simulink model "hexa_quaternion_FxTESO_ANSFT"  (R2023a)
settings: Solver=ode4  StartTime=0.0  StopTime=60  FixedStep=0.01  RelTol=1e-3
undefined symbols (not defined in the file or in its folder): F, Light, MIL
libraries: sharedtransform x9, dspsrcs4 x9, aerolibutil x8, simulink x5, sharedutil x3, simulink_extras x3, matrix_library x2, robotcorelib x1, aerolibwind2 x1, uavutilslib x1
(part 2 of 2)

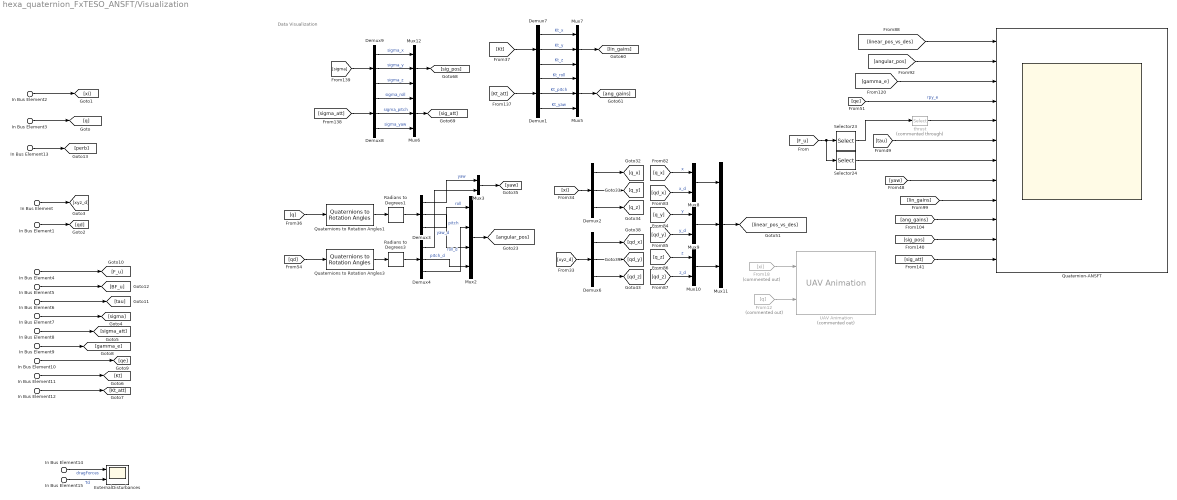
== system hexa_quaternion_FxTESO_ANSFT/Visualization ==
  note: Data Visualization
  In Bus Element2 : Inport  PortName=gamma_eta  Element=x
  In Bus Element3 : Inport  PortName=gamma_eta  Element=q
  In Bus Element13 : Inport  PortName=gamma_eta  Element=perb
  In Bus Element : Inport  Port=2  PortName=gamma_eta_d  Element=xyz_d
  In Bus Element1 : Inport  Port=2  PortName=gamma_eta_d  Element=qd
  In Bus Element4 : Inport  Port=3  PortName=u  Element=F_u
  In Bus Element5 : Inport  Port=3  PortName=u  Element=B-F_u
  In Bus Element6 : Inport  Port=3  PortName=u  Element=tau
  In Bus Element7 : Inport  Port=3  PortName=u  Element=sigma
  In Bus Element8 : Inport  Port=3  PortName=u  Element=sigma_att
  In Bus Element9 : Inport  Port=3  PortName=u  Element=gamma_e
  In Bus Element10 : Inport  Port=3  PortName=u  Element=eta_e
  In Bus Element11 : Inport  Port=3  PortName=u  Element=Kt
  In Bus Element12 : Inport  Port=3  PortName=u  Element=Kt_att
  In Bus Element14 : Inport  Port=4  PortName=perb  Element=perb
  In Bus Element15 : Inport  Port=4  PortName=perb  Element=Td
  Demux{1..4,6..9} (8 alike) : Demux  Outputs=3
  ExternalDisturbances : Scope  NumInputPorts=2
  From12 : From  Commented=on  GotoTag=q
  From18 : From  Commented=on  GotoTag=xi
  Mux{3,8..10} (4 alike) : Mux  Inputs=2
  Mux{5..7,11..12} (5 alike) : Mux  Inputs=3
  Mux2 : Mux
  Quaternion-ANSFT : Scope  NumInputPorts=12
  Quaternions to Rotation Angles1 : sharedtransform/Quaternions to Rotation Angles  rotationOrder=ZYX  aMode=aMode
  Quaternions to Rotation Angles3 : sharedtransform/Quaternions to Rotation Angles  rotationOrder=ZYX  aMode=aMode
  Radians to Degrees1 : simulink_extras/Transformations/Radians to Degrees
  Radians to Degrees3 : simulink_extras/Transformations/Radians to Degrees
  Selector23 : Selector  InputPortWidth=3  IndexOptions=Index vector (dialog)  Indices=[3]  OutputSizes=1
  Selector24 : Selector  InputPortWidth=3  IndexOptions=Index vector (dialog)  Indices=[1:2]  OutputSizes=1
  UAV Animation : uavutilslib/UAV Animation  Commented=on  UAVType=Multirotor  UAVSize=1  InertialZDirection=Down  SampleTime=-1
  thrust : Selector  Commented=through  InputPortWidth=3  IndexOptions=Index vector (dialog)  Indices=[3]  OutputSizes=1
  wires:
  [sigma_att] -> Demux8/1
  Radians to Degrees1/1 -> Demux3/1
  Demux3/3 -> Mux2/1  "roll"
  [lin_gains] -> Quaternion-ANSFT/9
  Mux11/1 -> [linear_pos_vs_des]
  [qe] -> Quaternion-ANSFT/4  "rpy_e"
  Mux3/1 -> [yaw]
  Demux6/1 -> [qd_x]
  Demux9/2 -> Mux12/2  "sigma_y"
  [yaw] -> Quaternion-ANSFT/8
  Mux5/1 -> [ang_gains]
  Mux10/1 -> Mux11/3
  Demux1/1 -> Mux5/1  "Kt_roll"
  Demux7/3 -> Mux7/3  "Kt_z"
  From12/1 -> UAV Animation/2
  [q_z] -> Mux10/1  "z"
  [linear_pos_vs_des] -> Quaternion-ANSFT/1
  Quaternions to Rotation Angles1/1 -> Radians to Degrees1/1
  [Kt] -> Demux7/1
  Demux4/2 -> Mux2/4  "pitch_d"
  Demux7/1 -> Mux7/1  "Kt_x"
  [qd] -> Quaternions to Rotation Angles3/1
  [qd_x] -> Mux8/2  "x_d"
  Demux7/2 -> Mux7/2  "Kt_y"
  Mux7/1 -> [lin_gains]
  Demux8/3 -> Mux6/3  "sigma_yaw"
  Demux6/2 -> [qd_y]
  [xyz_d] -> Demux6/1
  [gamma_e] -> Quaternion-ANSFT/3
  [sig_att] -> Quaternion-ANSFT/12
  [F_u] -> Selector24/1, Selector23/1
  Demux4/1 -> Mux3/2  "yaw_d"
  Selector24/1 -> Quaternion-ANSFT/7
  [q_x] -> Mux8/1  "x"
  [ang_gains] -> Quaternion-ANSFT/10
  Demux1/3 -> Mux5/3  "Kt_yaw"
  Mux9/1 -> Mux11/2
  Selector23/1 -> thrust/1
  Demux2/3 -> [q_z]
  Mux8/1 -> Mux11/1
  Demux3/1 -> Mux3/1  "yaw"
  [sig_pos] -> Quaternion-ANSFT/11
  [tau] -> Quaternion-ANSFT/6
  From18/1 -> UAV Animation/1
  Quaternions to Rotation Angles3/1 -> Radians to Degrees3/1
  Demux6/3 -> [qd_z]
  [q] -> Quaternions to Rotation Angles1/1
  Radians to Degrees3/1 -> Demux4/1
  [qd_z] -> Mux10/2  "z_d"
  Demux1/2 -> Mux5/2  "Kt_pitch"
  [qd_y] -> Mux9/2  "y_d"
  thrust/1 -> Quaternion-ANSFT/5
  Mux12/1 -> [sig_pos]
  Mux6/1 -> [sig_att]
  Demux2/2 -> [q_y]
  [sigma] -> Demux9/1
  Demux9/3 -> Mux12/3  "sigma_z"
  [q_y] -> Mux9/1  "y"
  Demux8/2 -> Mux6/2  "sigma_pitch"
  Demux2/1 -> [q_x]
  [Kt_att] -> Demux1/1
  Demux3/2 -> Mux2/3  "pitch"
  Mux2/1 -> [angular_pos]
  Demux9/1 -> Mux12/1  "sigma_x"
  Demux8/1 -> Mux6/1  "sigma_roll"
  [xi] -> Demux2/1
  [angular_pos] -> Quaternion-ANSFT/2
  Demux4/3 -> Mux2/2  "roll_d"
  In Bus Element3/1 -> [q]
  In Bus Element2/1 -> [xi]
  In Bus Element1/1 -> [qd]
  In Bus Element/1 -> [xyz_d]
  In Bus Element6/1 -> [tau]
  In Bus Element7/1 -> [sigma]
  In Bus Element8/1 -> [sigma_att]
  In Bus Element9/1 -> [gamma_e]
  In Bus Element10/1 -> [qe]
  In Bus Element4/1 -> [F_u]
  In Bus Element5/1 -> [BF_u]
  In Bus Element11/1 -> [Kt]
  In Bus Element12/1 -> [Kt_att]
  In Bus Element13/1 -> [perb]
  In Bus Element14/1 -> ExternalDisturbances/1  "dragForces"
  In Bus Element15/1 -> ExternalDisturbances/2  "Td"

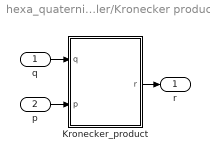
== system hexa_quaternion_FxTESO_ANSFT/Controller/Kronecker product4 ==
  q : Inport
  p : Inport  Port=2
  Kronecker_product : MATLAB Function  TreatAsAtomicUnit=on
  r : Outport
  wires:
  q/1 -> Kronecker_product/1(q)
  p/1 -> Kronecker_product/2(p)
  Kronecker_product/1(r) -> r/1

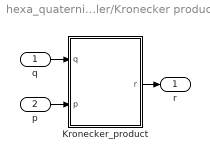
== system hexa_quaternion_FxTESO_ANSFT/Controller/Kronecker product6 ==
  q : Inport
  p : Inport  Port=2
  Kronecker_product : MATLAB Function  TreatAsAtomicUnit=on
  r : Outport
  wires:
  q/1 -> Kronecker_product/1(q)
  p/1 -> Kronecker_product/2(p)
  Kronecker_product/1(r) -> r/1

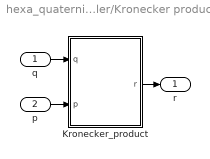
== system hexa_quaternion_FxTESO_ANSFT/Controller/Kronecker product7 ==
  q : Inport
  p : Inport  Port=2
  Kronecker_product : MATLAB Function  TreatAsAtomicUnit=on
  r : Outport
  wires:
  q/1 -> Kronecker_product/1(q)
  p/1 -> Kronecker_product/2(p)
  Kronecker_product/1(r) -> r/1

== system hexa_quaternion_FxTESO_ANSFT/Controller/quaterniontoPRV ==
  q : Inport
  MATLAB Function : MATLAB Function  TreatAsAtomicUnit=on
  lnq : Outport
  wires:
  MATLAB Function/1(lnq) -> lnq/1
  q/1 -> MATLAB Function/1(q)

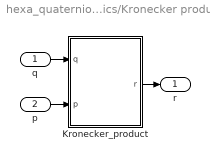
== system hexa_quaternion_FxTESO_ANSFT/Dynamics/Kronecker product ==
  q : Inport
  p : Inport  Port=2
  Kronecker_product : MATLAB Function  TreatAsAtomicUnit=on
  r : Outport
  wires:
  q/1 -> Kronecker_product/1(q)
  p/1 -> Kronecker_product/2(p)
  Kronecker_product/1(r) -> r/1

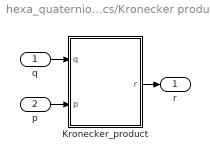
== system hexa_quaternion_FxTESO_ANSFT/Dynamics/Kronecker product1 ==
  q : Inport
  p : Inport  Port=2
  Kronecker_product : MATLAB Function  TreatAsAtomicUnit=on
  r : Outport
  wires:
  q/1 -> Kronecker_product/1(q)
  p/1 -> Kronecker_product/2(p)
  Kronecker_product/1(r) -> r/1

== system hexa_quaternion_FxTESO_ANSFT/Dynamics/Kronecker product2 ==
  q : Inport
  p : Inport  Port=2
  Kronecker_product : MATLAB Function  TreatAsAtomicUnit=on
  r : Outport
  wires:
  q/1 -> Kronecker_product/1(q)
  p/1 -> Kronecker_product/2(p)
  Kronecker_product/1(r) -> r/1

== system hexa_quaternion_FxTESO_ANSFT/Quaternion Observer/Kronecker product ==
  q : Inport
  p : Inport  Port=2
  Kronecker_product : MATLAB Function  TreatAsAtomicUnit=on
  r : Outport
  wires:
  q/1 -> Kronecker_product/1(q)
  p/1 -> Kronecker_product/2(p)
  Kronecker_product/1(r) -> r/1

== system hexa_quaternion_FxTESO_ANSFT/Quaternion Observer/Kronecker product1 ==
  q : Inport
  p : Inport  Port=2
  Kronecker_product : MATLAB Function  TreatAsAtomicUnit=on
  r : Outport
  wires:
  q/1 -> Kronecker_product/1(q)
  p/1 -> Kronecker_product/2(p)
  Kronecker_product/1(r) -> r/1

== system hexa_quaternion_FxTESO_ANSFT/Quaternion Observer/Kronecker product2 ==
  q : Inport
  p : Inport  Port=2
  Kronecker_product : MATLAB Function  TreatAsAtomicUnit=on
  r : Outport
  wires:
  q/1 -> Kronecker_product/1(q)
  p/1 -> Kronecker_product/2(p)
  Kronecker_product/1(r) -> r/1

== system hexa_quaternion_FxTESO_ANSFT/Quaternion Observer/Kronecker product3 ==
  q : Inport
  p : Inport  Port=2
  Kronecker_product : MATLAB Function  TreatAsAtomicUnit=on
  r : Outport
  wires:
  q/1 -> Kronecker_product/1(q)
  p/1 -> Kronecker_product/2(p)
  Kronecker_product/1(r) -> r/1

== system hexa_quaternion_FxTESO_ANSFT/Reference/Kronecker product3 ==
  q : Inport
  p : Inport  Port=2
  Kronecker_product : MATLAB Function  TreatAsAtomicUnit=on
  r : Outport
  wires:
  q/1 -> Kronecker_product/1(q)
  p/1 -> Kronecker_product/2(p)
  Kronecker_product/1(r) -> r/1

== system hexa_quaternion_FxTESO_ANSFT/Reference/Kronecker product5 ==
  q : Inport
  p : Inport  Port=2
  Kronecker_product : MATLAB Function  TreatAsAtomicUnit=on
  r : Outport
  wires:
  q/1 -> Kronecker_product/1(q)
  p/1 -> Kronecker_product/2(p)
  Kronecker_product/1(r) -> r/1

== matlab function hexa_quaternion_FxTESO_ANSFT/Quaternion Observer/calculateCvMatrix ==
  data: q input; Cv output
function Cv = fcn(q)

q0 = q(1);
q1 = q(2);
q2 = q(3);
q3 = q(4);

Cv = [q0, -q3, q2;
      q3, q0, -q1;
      -q2, q1, q0] * 0.5;

Cv = pinv(Cv);

== matlab function hexa_quaternion_FxTESO_ANSFT/Reference/Kronecker product3/Kronecker_product ==
  data: q input; r output size=[4 1]; p input
function r = fcn(q, p)

%{
    Function to describe in matrix math the Kronecker product between
    two quaternions
    
    r = p kronecker q
    %}

    len = length(p);

    if len == 3 && length(q) == 4
        p1 = [0; p];
        q0 = q(1);
        q1 = q(2);
        q2 = q(3);
        q3 = q(4);
        
        % skew symmetric matrix
        q_matrix = [q0, -q1, -q2, -q3;
                  q1, q0, -q3, q2;
                  q2, q3, q0, -q1;
                  q3, -q2, q1, q0];
        
        r = q_matrix * p1;

    elseif len == 4
        q0 = q(1);
        q1 = q(2);
        q2 = q(3);
        q3 = q(4);
        
        % skew symmetric matrix
        q_matrix = [q0, -q1, -q2, -q3;
                  q1, q0, -q3, q2;
                  q2, q3, q0, -q1;
                  q3, -q2, q1, q0];
        
        r = q_matrix * p;

    else
        error('Quaternions dimensions do not match')
    end

== matlab function hexa_quaternion_FxTESO_ANSFT/Controller/quaterniontoPRV/MATLAB Function ==
  data: q input; lnq output size=[3 1]
function lnq = fcn(q)

if length(q) == 4
    q0 = q(1);
    q_vec = [q(2); q(3); q(4)];

    if norm(q_vec) == 0
        lnq = [0; 0; 0];
    else
        % q0 = real(q0);
        lnq = (q_vec / (norm(q_vec)) ) * acos(q0);
    end
else
    error('Input must be a vector 4 by 1 (Quaternion)')
end

== matlab function hexa_quaternion_FxTESO_ANSFT/Reference/calculateAttitudeTrajectory ==
  data: qx output; qy output; t input; qz output; w_d output; w_d_dot output
function [qx, qy, qz, w_d, w_d_dot] = fcn(t)

roll = 0.0;
pitch = 0.0;
% yaw = 0;
% w_d = [0; 0; 0];

if t < 5
    % roll = 0;
    % roll_d = 0;
    % pitch = 0;
    yaw = 0;
    w_d = [0; 0; 0];
else
    % roll = 5 * pi / 180 * sin(t - 5);
    % roll_d = 5 * pi / 180 * cos(t - 5);
    yaw = 5 * pi * (t - 5) / 180;
    w_d = [0; 0; 5 * pi / 180];
    % w_d = [0; 0; 0];
    % w_d = [roll_d; 0; 0];
end

qx = [cos(roll/2);
      sin(roll/2);
      0;
      0];

qy = [cos(pitch/2);
      0;
      sin(pitch/2);
      0];

qz = [cos(yaw/2);
      0;
      0;
      sin(yaw/2)];

% w_d = [0; 0; 0];
w_d_dot = [0; 0; 0];

== matlab function hexa_quaternion_FxTESO_ANSFT/Controller/Kronecker product4/Kronecker_product ==
  data: q input; r output size=[4 1]; p input
function r = fcn(q, p)

%{
    Function to describe in matrix math the Kronecker product between
    two quaternions
    
    r = p kronecker q
    %}

    len = length(p);

    if len == 3 && length(q) == 4
        p1 = [0; p];
        q0 = q(1);
        q1 = q(2);
        q2 = q(3);
        q3 = q(4);
        
        % skew symmetric matrix
        q_matrix = [q0, -q1, -q2, -q3;
                  q1, q0, -q3, q2;
                  q2, q3, q0, -q1;
                  q3, -q2, q1, q0];
        
        r = q_matrix * p1;

    elseif len == 4
        q0 = q(1);
        q1 = q(2);
        q2 = q(3);
        q3 = q(4);
        
        % skew symmetric matrix
        q_matrix = [q0, -q1, -q2, -q3;
                  q1, q0, -q3, q2;
                  q2, q3, q0, -q1;
                  q3, -q2, q1, q0];
        
        r = q_matrix * p;

    else
        error('Quaternions dimensions do not match')
    end

== matlab function hexa_quaternion_FxTESO_ANSFT/Controller/ANSFT parameters ==
  data: xi1 output; xi2 output; lambda1 output; unused input; lambda2 output; alpha output; beta output
function [xi1, xi2, lambda1, lambda2, alpha, beta] = fcn(~)

%% Constantes de la Superficie deslizante
% zeta1 parecido a una ganancia proporcional
xi1 = [2.5; 2.5; 1.5; 1; 1; 1];
%zeta2 parecido a una ganancia derivatida
xi2 = [1.25; 1.25; 2; 0.5; 0.5; 0.5];
% lambda 1 > lambda2
lambda1 = [1.5; 1.5; 1.75; 2; 2; 2];
% 1 < lambda2 < 2
lambda2 = [1.2; 1.2; 1.25; 1.2; 1.2; 1.2];
%% Constantes del control auxiliar
%minimize sigma
alpha = [1.75; 1.75; 0.625; 2.5; 2.5; 1.25];
%aumetnar control, aumentar energía del sistema
beta = [2.5; 2.5; 0.1; 0.05; 0.05; 0.25];

== matlab function hexa_quaternion_FxTESO_ANSFT/Controller/Kronecker product6/Kronecker_product ==
  data: q input; r output; p input
function r = fcn(q, p)

%{
    Function to describe in matrix math the Kronecker product between
    two quaternions
    
    r = p kronecker q
    %}

    len = length(p);

    if len == 3
        p1 = [0; p];
        q0 = q(1);
        q1 = q(2);
        q2 = q(3);
        q3 = q(4);
        
        % skew symmetric matrix
        q_matrix = [q0, -q1, -q2, -q3;
                  q1, q0, -q3, q2;
                  q2, q3, q0, -q1;
                  q3, -q2, q1, q0];
        
        r = q_matrix * p1;

    elseif len == 4
        q0 = q(1);
        q1 = q(2);
        q2 = q(3);
        q3 = q(4);
        
        % skew symmetric matrix
        q_matrix = [q0, -q1, -q2, -q3;
                  q1, q0, -q3, q2;
                  q2, q3, q0, -q1;
                  q3, -q2, q1, q0];
        
        r = q_matrix * p;

    else
        error('Quaternions dimensions do not match')
    end

== matlab function hexa_quaternion_FxTESO_ANSFT/Controller/Kronecker product7/Kronecker_product ==
  data: q input; r output; p input
function r = fcn(q, p)

%{
    Function to describe in matrix math the Kronecker product between
    two quaternions
    
    r = p kronecker q
    %}

    len = length(p);

    if len == 3
        p1 = [0; p];
        q0 = q(1);
        q1 = q(2);
        q2 = q(3);
        q3 = q(4);
        
        % skew symmetric matrix
        q_matrix = [q0, -q1, -q2, -q3;
                  q1, q0, -q3, q2;
                  q2, q3, q0, -q1;
                  q3, -q2, q1, q0];
        
        r = q_matrix * p1;

    elseif len == 4
        q0 = q(1);
        q1 = q(2);
        q2 = q(3);
        q3 = q(4);
        
        % skew symmetric matrix
        q_matrix = [q0, -q1, -q2, -q3;
                  q1, q0, -q3, q2;
                  q2, q3, q0, -q1;
                  q3, -q2, q1, q0];
        
        r = q_matrix * p;

    else
        error('Quaternions dimensions do not match')
    end

== matlab function hexa_quaternion_FxTESO_ANSFT/Quaternion Observer/FxTESO Constants ==
  data: epsilon1 output; epsilon2 output; epsilon3 output; epsilon4 output; mu1 output; mu2 output; mu3 output; alpha output; beta output
function [epsilon1, epsilon2, epsilon3, epsilon4, mu1, mu2, mu3, alpha, beta] = fcn

epsilon1 = [16; 16; 16];
epsilon2 = [60; 60; 60];
epsilon3 = [100; 100; 100];

epsilon4 = [0.01, 0.01, 0.01]';

mu1 = epsilon1;
mu2 = epsilon2;
mu3 = epsilon3;

alpha = [0.6; 0.6; 0.6];

beta = [1.2; 1.2; 1.2];

== matlab function hexa_quaternion_FxTESO_ANSFT/Quaternion Observer/calculateActuationMatrix ==
  data: pose input; B output
function B  = fcn(pose)

roll = pose(4);
pitch = pose(5);
yaw = pose(6);

R1 = [cos(yaw)*cos(pitch), -cos(roll)*sin(yaw) + cos(yaw)*sin(roll)*sin(pitch), sin(roll)*sin(yaw) + cos(roll)*cos(yaw)*sin(pitch);
       cos(pitch)*sin(yaw), cos(roll)*cos(yaw) + sin(yaw)*sin(pitch)*sin(roll), -cos(yaw)*sin(roll) + sin(yaw)*sin(pitch)*cos(roll);
       -sin(pitch), cos(pitch)*sin(roll), cos(pitch)*cos(roll)];

R2 = [1, sin(roll)*tan(pitch), cos(roll)*tan(pitch);
      0, cos(roll), -sin(roll);
      0, sin(roll)/cos(pitch), cos(roll)/cos(pitch)];

Rzeros = zeros(3);

% B = [transpose(R1), Rzeros;
%      Rzeros, inv(R2)];

B = [R1, Rzeros;
     Rzeros, R2];

== matlab function hexa_quaternion_FxTESO_ANSFT/Quaternion Observer/Kronecker product/Kronecker_product ==
  data: q input; r output size=[4 1]; p input
function r = fcn(q, p)

%{
    Function to describe in matrix math the Kronecker product between
    two quaternions
    
    r = p kronecker q
    %}

    len = length(p);

    if len == 3 && length(q) == 4
        p1 = [0; p];
        q0 = q(1);
        q1 = q(2);
        q2 = q(3);
        q3 = q(4);
        
        % skew symmetric matrix
        q_matrix = [q0, -q1, -q2, -q3;
                  q1, q0, -q3, q2;
                  q2, q3, q0, -q1;
                  q3, -q2, q1, q0];
        
        r = q_matrix * p1;

    elseif len == 4
        q0 = q(1);
        q1 = q(2);
        q2 = q(3);
        q3 = q(4);
        
        % skew symmetric matrix
        q_matrix = [q0, -q1, -q2, -q3;
                  q1, q0, -q3, q2;
                  q2, q3, q0, -q1;
                  q3, -q2, q1, q0];
        
        r = q_matrix * p;

    else
        error('Quaternions dimensions do not match')
    end

== matlab function hexa_quaternion_FxTESO_ANSFT/Quaternion Observer/Kronecker product1/Kronecker_product ==
  data: q input; r output size=[4 1]; p input
function r = fcn(q, p)

%{
    Function to describe in matrix math the Kronecker product between
    two quaternions
    
    r = p kronecker q
    %}

    len = length(p);

    if len == 3 && length(q) == 4
        p1 = [0; p];
        q0 = q(1);
        q1 = q(2);
        q2 = q(3);
        q3 = q(4);
        
        % skew symmetric matrix
        q_matrix = [q0, -q1, -q2, -q3;
                  q1, q0, -q3, q2;
                  q2, q3, q0, -q1;
                  q3, -q2, q1, q0];
        
        r = q_matrix * p1;

    elseif len == 4
        q0 = q(1);
        q1 = q(2);
        q2 = q(3);
        q3 = q(4);
        
        % skew symmetric matrix
        q_matrix = [q0, -q1, -q2, -q3;
                  q1, q0, -q3, q2;
                  q2, q3, q0, -q1;
                  q3, -q2, q1, q0];
        
        r = q_matrix * p;

    else
        error('Quaternions dimensions do not match')
    end

== matlab function hexa_quaternion_FxTESO_ANSFT/Turbulence Model/ExternalDisturbanceTorques ==
  data: t input; Td output
function Td = fcn(t)

Td = [0.005 * sin(0.1  * t);
      0.005 * sin(0.2 * t);
      0.005 * cos(0.2 * t)];

== matlab function hexa_quaternion_FxTESO_ANSFT/Quaternion Observer/Kronecker product2/Kronecker_product ==
  data: q input; r output size=[4 1]; p input
function r = fcn(q, p)

%{
    Function to describe in matrix math the Kronecker product between
    two quaternions
    
    r = p kronecker q
    %}

    len = length(p);

    if len == 3 && length(q) == 4
        p1 = [0; p];
        q0 = q(1);
        q1 = q(2);
        q2 = q(3);
        q3 = q(4);
        
        % skew symmetric matrix
        q_matrix = [q0, -q1, -q2, -q3;
                  q1, q0, -q3, q2;
                  q2, q3, q0, -q1;
                  q3, -q2, q1, q0];
        
        r = q_matrix * p1;

    elseif len == 4
        q0 = q(1);
        q1 = q(2);
        q2 = q(3);
        q3 = q(4);
        
        % skew symmetric matrix
        q_matrix = [q0, -q1, -q2, -q3;
                  q1, q0, -q3, q2;
                  q2, q3, q0, -q1;
                  q3, -q2, q1, q0];
        
        r = q_matrix * p;

    else
        error('Quaternions dimensions do not match')
    end

== matlab function hexa_quaternion_FxTESO_ANSFT/Quaternion Observer/Kronecker product3/Kronecker_product ==
  data: q input; r output size=[4 1]; p input
function r = fcn(q, p)

%{
    Function to describe in matrix math the Kronecker product between
    two quaternions
    
    r = p kronecker q
    %}

    len = length(p);

    if len == 3 && length(q) == 4
        p1 = [0; p];
        q0 = q(1);
        q1 = q(2);
        q2 = q(3);
        q3 = q(4);
        
        % skew symmetric matrix
        q_matrix = [q0, -q1, -q2, -q3;
                  q1, q0, -q3, q2;
                  q2, q3, q0, -q1;
                  q3, -q2, q1, q0];
        
        r = q_matrix * p1;

    elseif len == 4
        q0 = q(1);
        q1 = q(2);
        q2 = q(3);
        q3 = q(4);
        
        % skew symmetric matrix
        q_matrix = [q0, -q1, -q2, -q3;
                  q1, q0, -q3, q2;
                  q2, q3, q0, -q1;
                  q3, -q2, q1, q0];
        
        r = q_matrix * p;

    else
        error('Quaternions dimensions do not match')
    end

== matlab function hexa_quaternion_FxTESO_ANSFT/Quaternion Observer/FxTQESO Constants ==
  data: epsilon1 output; epsilon2 output; epsilon3 output; epsilon4 output; mu1 output; mu2 output; mu3 output; alpha output; beta output
function [epsilon1, epsilon2, epsilon3, epsilon4, mu1, mu2, mu3, alpha, beta] = fcn

epsilon1 = [16; 16; 16];
epsilon2 = [150; 150; 150];
epsilon3 = [450; 450; 450];

epsilon4 = [0.01, 0.01, 0.01]';

mu1 = epsilon1;
mu2 = epsilon2;
mu3 = epsilon3;

alpha = [0.6; 0.6; 0.6];

beta = [1.2; 1.2; 1.2];

== matlab function hexa_quaternion_FxTESO_ANSFT/Subsystem/MATLAB Function ==
  data: q input; lnq output size=[3 1]
function lnq = fcn(q)

if length(q) == 4
    q0 = q(1);
    
    q_vec = [q(2); q(3); q(4)];

    if norm(q_vec) == 0
        lnq = [0; 0; 0];
    else
        lnq = (q_vec / (norm(q_vec)) ) * acos(q0);
    end
else
    error('Input must be a vector 4 by 1 (Quaternion)')
end

== matlab function hexa_quaternion_FxTESO_ANSFT/Dynamics/Kronecker product/Kronecker_product ==
  data: q input; r output size=[4 1]; p input
function r = fcn(q, p)

%{
    Function to describe in matrix math the Kronecker product between
    two quaternions
    
    r = p kronecker q
    %}

    len = length(p);

    if len == 3 && length(q) == 4
        p1 = [0; p];
        q0 = q(1);
        q1 = q(2);
        q2 = q(3);
        q3 = q(4);
        
        % skew symmetric matrix
        q_matrix = [q0, -q1, -q2, -q3;
                  q1, q0, -q3, q2;
                  q2, q3, q0, -q1;
                  q3, -q2, q1, q0];
        
        r = q_matrix * p1;

    elseif len == 4
        q0 = q(1);
        q1 = q(2);
        q2 = q(3);
        q3 = q(4);
        
        % skew symmetric matrix
        q_matrix = [q0, -q1, -q2, -q3;
                  q1, q0, -q3, q2;
                  q2, q3, q0, -q1;
                  q3, -q2, q1, q0];
        
        r = q_matrix * p;

    else
        error('Quaternions dimensions do not match')
    end

== matlab function hexa_quaternion_FxTESO_ANSFT/Dynamics/Constants Functions ==
  data: J output; m output; g output
function [J, m, g] = fcn

m = 1.8; % kg

Jxx =  0.0411; % kg m²
Jyy = 0.0478; % kg m²
Jzz = 0.0599; % kg m²

J = [Jxx, 0, 0;
     0, Jyy, 0;
     0, 0, Jzz];

g = [0; 0; -9.81];

== matlab function hexa_quaternion_FxTESO_ANSFT/norm ==
  data: u input; y output
function y = fcn(u)

y = norm(u);

== matlab function hexa_quaternion_FxTESO_ANSFT/Dynamics/Kronecker product1/Kronecker_product ==
  data: q input; r output; p input
function r = fcn(q, p)

%{
    Function to describe in matrix math the Kronecker product between
    two quaternions
    
    r = p kronecker q
    %}

    len = length(p);

    if len == 3
        p1 = [0; p];
        q0 = q(1);
        q1 = q(2);
        q2 = q(3);
        q3 = q(4);
        
        % skew symmetric matrix
        q_matrix = [q0, -q1, -q2, -q3;
                  q1, q0, -q3, q2;
                  q2, q3, q0, -q1;
                  q3, -q2, q1, q0];
        
        r = q_matrix * p1;

    elseif len == 4
        q0 = q(1);
        q1 = q(2);
        q2 = q(3);
        q3 = q(4);
        
        % skew symmetric matrix
        q_matrix = [q0, -q1, -q2, -q3;
                  q1, q0, -q3, q2;
                  q2, q3, q0, -q1;
                  q3, -q2, q1, q0];
        
        r = q_matrix * p;

    else
        error('Quaternions dimensions do not match')
    end

== matlab function hexa_quaternion_FxTESO_ANSFT/Dynamics/Kronecker product2/Kronecker_product ==
  data: q input; r output; p input
function r = fcn(q, p)

%{
    Function to describe in matrix math the Kronecker product between
    two quaternions
    
    r = p kronecker q
    %}

    len = length(p);

    if len == 3
        p1 = [0; p];
        q0 = q(1);
        q1 = q(2);
        q2 = q(3);
        q3 = q(4);
        
        % skew symmetric matrix
        q_matrix = [q0, -q1, -q2, -q3;
                  q1, q0, -q3, q2;
                  q2, q3, q0, -q1;
                  q3, -q2, q1, q0];
        
        r = q_matrix * p1;

    elseif len == 4
        q0 = q(1);
        q1 = q(2);
        q2 = q(3);
        q3 = q(4);
        
        % skew symmetric matrix
        q_matrix = [q0, -q1, -q2, -q3;
                  q1, q0, -q3, q2;
                  q2, q3, q0, -q1;
                  q3, -q2, q1, q0];
        
        r = q_matrix * p;

    else
        error('Quaternions dimensions do not match')
    end

== matlab function hexa_quaternion_FxTESO_ANSFT/Reference/Kronecker product5/Kronecker_product ==
  data: q input; r output size=[4 1]; p input
function r = fcn(q, p)

%{
    Function to describe in matrix math the Kronecker product between
    two quaternions
    
    r = p kronecker q
    %}

    len = length(p);

    if len == 3 && length(q) == 4
        p1 = [0; p];
        q0 = q(1);
        q1 = q(2);
        q2 = q(3);
        q3 = q(4);
        
        % skew symmetric matrix
        q_matrix = [q0, -q1, -q2, -q3;
                  q1, q0, -q3, q2;
                  q2, q3, q0, -q1;
                  q3, -q2, q1, q0];
        
        r = q_matrix * p1;

    elseif len == 4
        q0 = q(1);
        q1 = q(2);
        q2 = q(3);
        q3 = q(4);
        
        % skew symmetric matrix
        q_matrix = [q0, -q1, -q2, -q3;
                  q1, q0, -q3, q2;
                  q2, q3, q0, -q1;
                  q3, -q2, q1, q0];
        
        r = q_matrix * p;

    else
        error('Quaternions dimensions do not match')
    end

== matlab function hexa_quaternion_FxTESO_ANSFT/Reference/Helicoidal Trajectory ==
  data: time input; pose_d output; pose_d_dot output; pose_d_ddot output
function [pose_d, pose_d_dot, pose_d_ddot]= fcn(time)

% pos_z = time / 12;
f = 0.15;
arg = f * (time - 5);
r = 2;

% hover for 5 s | include inclination in roll
% 5 metros al menos

if (time < 5)
    pos_x = 0;
    pos_y = 0;
    % roll = 0;
    pos_z = 0.4 * time;
else
    pos_x = -r + r * cos (arg);
    pos_y = r * sin (arg);
    pos_z = 2;
end

% roll = 0;
% yaw = time * 0;

pose_d = [pos_x;
          pos_y;
          pos_z];
          % roll;
          % 0;
          % yaw];

% pos_z_dot = 1 / 12;

% hover for 5 s
if (time < 5)
    pos_x_dot = 0;
    pos_y_dot = 0;
    pos_z_dot = 0.4;
else
    pos_x_dot = - f * r * sin(arg);
    pos_y_dot = f * r * cos(arg);
    pos_z_dot= 0;
end

% yaw_dot = 0;

pose_d_dot = [pos_x_dot;
              pos_y_dot;
              pos_z_dot];
              % 0;
              % 0;
              % yaw_dot];

pos_z_ddot = 0;
% hover for 5 s
if (time < 5)
    pos_x_ddot = 0;
    pos_y_ddot = 0;
else
    pos_x_ddot = - f * f * r * cos(arg);
    pos_y_ddot = - f * f * r * sin(arg);
end

% yaw_ddot = 0;

pose_d_ddot = [pos_x_ddot;
               pos_y_ddot;
               pos_z_ddot];
               % 0;
               % 0;
               % yaw_ddot];

== matlab function hexa_quaternion_FxTESO_ANSFT/Reference/Lemniscate Trajectory ==
  data: time input; pose_d output; pose_d_dot output; pose_d_ddot output
function [pose_d, pose_d_dot, pose_d_ddot]= fcn(time)

%% Positions

arg = time / 4;

pos_x = cos(arg) ./ (1 + sin(arg) .* sin(arg));
pos_y = cos(arg) .* sin(arg) ./ (1 + sin(arg) .* sin(arg));
pos_z = sin(arg);

% yaw = time * 0;

pose_d = [pos_x;
          pos_y;
          pos_z];
          % 0;
          % 0;
          % yaw];

%% Velocities

pos_z_dot = 0.25 * cos(arg);
pos_x_dot = - sin(arg)/(4*(sin(arg)^2 + 1)) - (cos(arg)^2*sin(arg))/(2*(sin(arg)^2 + 1)^2);
pos_y_dot = cos(arg)^2/(4*(sin(arg)^2 + 1)) - sin(arg)^2/(4*(sin(arg)^2 + 1)) - (cos(arg)^2*sin(arg)^2)/(2*(sin(arg)^2 + 1)^2);
% yaw_dot = 0;

pose_d_dot = [pos_x_dot;
              pos_y_dot;
              pos_z_dot];
              % 0;
              % 0;
              % yaw_dot];

%% Accelerations

pos_z_ddot = -0.25 * 0.25 * sin(arg);
pos_x_ddot = 0;
pos_y_ddot = 0;
% yaw_ddot = 0;

pose_d_ddot = [pos_x_ddot;
               pos_y_ddot;
               pos_z_ddot];
               % 0;
               % 0;
               % yaw_ddot];

== matlab function hexa_quaternion_FxTESO_ANSFT/Controller/calculatePWM ==
  data: omega2 input; pwm output
function pwm = fcn(omega2)

pwm = -1.3121e-09 .* omega2 .* omega2 + 0.00208 .* omega2 + 1107.922;
